simulink model "OCTAGONEngine_CMcoder"  (R2019b)
settings: Solver=ode1  StartTime=0.0  StopTime=inf  FixedStep=0.001  RelTol=1e-3
PreLoadFcn:
  | vehicle = 'Car'; if ~length(which('cmself')), run ../cmenv; end
  | OCTAGONEngine_CMcoder_bus
  | addpath ../../../../src/OCTAGONEngine
PostLoadFcn:
  | [StrFileName,StrPathName] = uigetfile('*.m','Select OCTAGONEngine Parameter File', "../../../../src/OCTAGONEngine");
  | if ~ischar(StrFileName)
  |   disp('User cancelled');
  |   return
  | end
  | StrFullPathName = fullfile(StrPathName, StrFileName);
  | run(StrFullPathName);
  | 
  | load_system ('mdl_OCTAGONEngine');
  | set_param('mdl_OCTAGONEngine/Engine Trq/Target torque to  Load Calculation/Engine Load Calculation/Transfer Fcn','Realization','general');
libraries: CarMaker4SL x10
Description:
  | CarMaker Plug-in Model Target
settings Model: TunableVars=DeadTime,ECU_D_Param,ECU_I_Param,ECU_P_Param,EngineDisturbanceMode,EngineTrq_off,Engine_negativeTrq,Engine_positiveTrq,Engine_rotv_negative,Engine_rotv_positive,ISC_I_Param,ISC_P_Param,NegativeTrq_Irregularity_ActivateFlag,TransferFn_Num  TunableVarsStorageClass=Auto,Auto,Auto,Auto,Auto,Auto,Auto,Auto,Auto,Auto,Auto,Auto,Auto,Auto  TunableVarsTypeQualifier=,,,,,,,,,,,,,  Creator=uib55286  LastModifiedBy=uib55286
settings RTWCC: Description=CarMaker Plug-in Model Target  SystemTargetFile=CarMaker.tlc  TemplateMakefile=CarMaker_unix-win64.tmf
settings CodeAppCC: MaxIdLength=127
settings STFCustomTargetCC: TargetLangStandard=C99 (ISO)  CombineOutputUpdateFcns=on  MultiInstanceERTCode=on  CodeInterfacePackaging=Reusable function  GenerateAllocFcn=on  SystemTargetFile=CarMaker.tlc
settings GRTTargetCC: ParMdlRefBuildCompliant=off  CompOptLevelCompliant=off  ConcurrentExecutionCompliant=off  MatFileLogging=off  MultiInstanceERTCode=on  CodeInterfacePackaging=Reusable function  CPPClassGenCompliant=off  GenerateAllocFcn=on  UseToolchainInfoCompliant=off  RTWCAPISignals=on  RTWCAPIParams=on  RTWCAPIStates=on

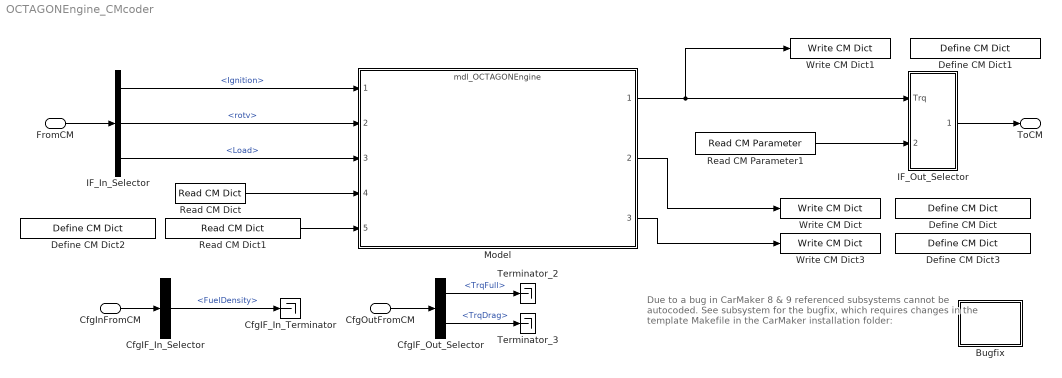
== system OCTAGONEngine_CMcoder ==
  note: Due to a bug in CarMaker 8 & 9 referenced subsystems cannot
      | be autocoded. See subsystem for the bugfix, which requires changes
      | in the template Makefile in the CarMaker installation folder:
  FromCM : Inport  OutDataTypeStr=Bus: cmPTEngineIn
  CfgInFromCM : Inport  Port=2  OutDataTypeStr=Bus: cmPTEngineCfgIn
  CfgOutFromCM : Inport  Port=3  OutDataTypeStr=Bus: cmPTEngineCfgOut
  Bugfix : Subsystem
  CfgIF_In_Selector : BusSelector  OutputSignals=FuelDensity
  CfgIF_In_Terminator : Terminator
  CfgIF_Out_Selector : BusSelector  OutputSignals=TrqFull,TrqDrag
  Define CM Dict : CarMaker4SL/Define CM Dict  xname=OCTAGONEngine.ECULoad  xmono=off  xtype=Double4  xdvaplace=None  xnstates=0  xfirststate=0  xinitial=0
  Define CM Dict1 : CarMaker4SL/Define CM Dict  xname=OCTAGONEngine.Torque  xunit=Nm  xmono=off  xtype=Double4  xdvaplace=None  xnstates=0  xfirststate=0  xinitial=0
  Define CM Dict2 : CarMaker4SL/Define CM Dict  xname=OCTAGONEngine.Trq_Trg  xunit=Nm  xmono=off  xtype=Double4  xdvaplace=IO_In  xnstates=0  xfirststate=0  xinitial=-9999
  Define CM Dict3 : CarMaker4SL/Define CM Dict  xname=OCTAGONEngine.rotv  xunit=rad/s  xmono=off  xtype=Double4  xdvaplace=None  xnstates=0  xfirststate=0  xinitial=0
  IF_In_Selector : BusSelector  OutputSignals=Ignition,rotv,Load
  IF_Out_Selector : Subsystem  mask(Signal Selection){}
      mask help: Signal Selection Block
      settings: OpenFcn=cmSignalSelect('SignalSelection_CB',gcb)
  Model : ModelReference  ModelNameDialog=mdl_OCTAGONEngine.slx  SimulationMode=Normal  ModelReferenceVersion=1.46
  Read CM Dict : CarMaker4SL/Read CM Dict  xname=Car.v  xsync=off
  Read CM Dict1 : CarMaker4SL/Read CM Dict  xname=OCTAGONEngine.Trq_Trg  xsync=off
  Read CM Parameter1 : CarMaker4SL/Read CM Parameter  xfile=Vehicle  xkey=PowerTrain.Engine.I  xnout=1  xdefaults=0.4  xmuxed=on
      settings: SourceProductName=CarMaker4SL
  Terminator_2 : Terminator
  Terminator_3 : Terminator
  Write CM Dict : CarMaker4SL/Write CM Dict  xname=OCTAGONEngine.ECULoad  xsync=off
  Write CM Dict1 : CarMaker4SL/Write CM Dict  xname=OCTAGONEngine.Torque  xsync=off
  Write CM Dict3 : CarMaker4SL/Write CM Dict  xname=OCTAGONEngine.rotv  xsync=off
  ToCM : Outport  OutDataTypeStr=Bus: cmPTEngineOut
  wires:
  FromCM/1 -> IF_In_Selector/1
  IF_Out_Selector/1(ToCM) -> ToCM/1
  CfgInFromCM/1 -> CfgIF_In_Selector/1
  CfgIF_In_Selector/1 -> CfgIF_In_Terminator/1  "<FuelDensity>"
  CfgOutFromCM/1 -> CfgIF_Out_Selector/1
  Model/1 -> IF_Out_Selector/1(Trq), Write CM Dict1/1
  Read CM Parameter1/1 -> IF_Out_Selector/2(Inert)
  IF_In_Selector/1 -> Model/1  "<Ignition>"
  IF_In_Selector/2 -> Model/2  "<rotv>"
  IF_In_Selector/3 -> Model/3  "<Load>"
  CfgIF_Out_Selector/1 -> Terminator_2/1  "<TrqFull>"
  CfgIF_Out_Selector/2 -> Terminator_3/1  "<TrqDrag>"
  Read CM Dict/1 -> Model/4
  Model/2 -> Write CM Dict/1
  Model/3 -> Write CM Dict3/1
  Read CM Dict1/1 -> Model/5

== system OCTAGONEngine_CMcoder/Bugfix ==
  note: 1) Open the following file with an editor:
      | <IPGHOME>\carmaker\win64-8.1.1\Matlab\R2019b\CarMaker_unix-win64.tmf
      |
      | 2) Search this location (apporx line 71-74):
      | OBJS = $(MODEL).o $(patsubst rt_malloc_main.o,,$(SRCS:.c=.o))
      | ifeq ($(MODELREF_TARGET_TYPE), NONE)
      | OBJS += $(WRAPPER).o
      | endif
      |
      | 3) Move '$(MODEL).o' in the if block:
      | OBJS = $(patsubst rt_malloc_main.o,,$(SRCS:.c=.o))
      | ifeq ($(MODELREF_TARGET_TYPE), NONE)
      | OBJS += $(MODEL).o $(WRAPPER).o
      | endif
      |
      | If you want to use another CM or Matlab version, please take into account that you have to adjust the path in step 1)

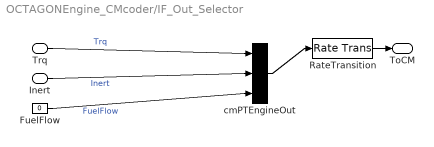
== system OCTAGONEngine_CMcoder/IF_Out_Selector ==
  Trq : Inport
  Inert : Inport  Port=2
  FuelFlow : Constant  Value=0
  RateTransition : RateTransition  OutPortSampleTime=str2num(get_param(bdroot,'FixedStep'))
  cmPTEngineOut : BusCreator  Inputs=3
  ToCM : Outport
  wires:
  RateTransition/1 -> ToCM/1
  cmPTEngineOut/1 -> RateTransition/1
  FuelFlow/1 -> cmPTEngineOut/3  "FuelFlow"
  Trq/1 -> cmPTEngineOut/1  "Trq"
  Inert/1 -> cmPTEngineOut/2  "Inert"
